simulink library "Adaptive_FaultTolerantControl"  (R2015a)
settings: Solver=ode45  StartTime=0.0  StopTime=10.0  RelTol=1e-3
libraries: qcatlib x1
settings Model: Creator=David  LastModifiedBy=David
settings OptimizationCC: ExpressionDepthLimit=2147483647
settings DebuggingCC: UnderspecifiedInitializationDetection=Classic  MergeDetectMultiDrivingBlocksExec=none  SolverPrmCheckMsg=warning  StateNameClashWarn=warning

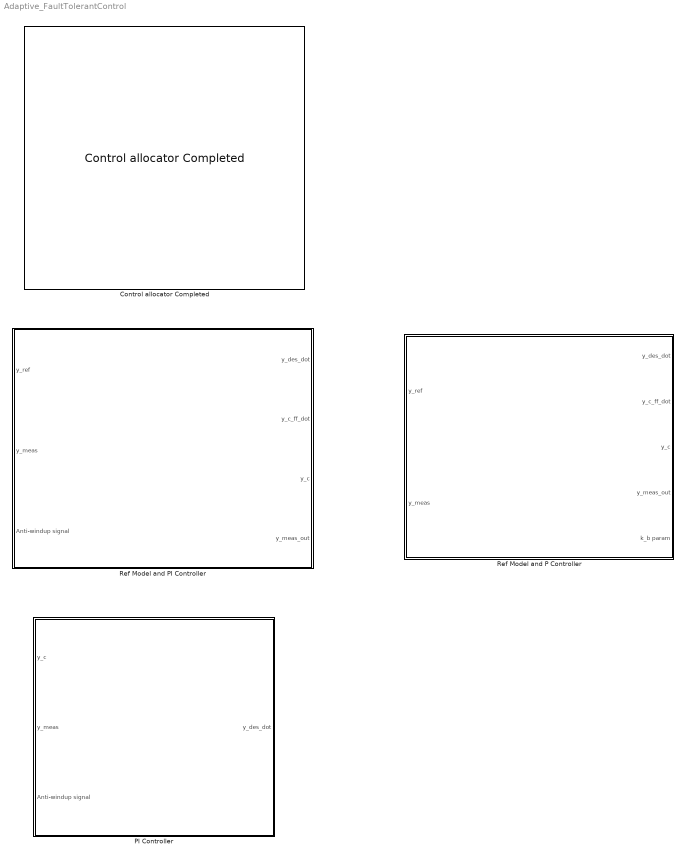
== system Adaptive_FaultTolerantControl ==
  "Control allocator Completed " : qcatlib/Control allocator Completed   alg=WLS  CA_type=DYN  iter_max=100  gamma=1e6  k_B=3  m_B=7  T=0.01  tol=0
  PI Controller : Subsystem  mask(PI Controller){delta=0, K_a=0, y_i=0, Des_way=auto, omega_n=10, xi=0.9, Z1=0, K_b=12, f_i=0.25, f_c=1}
      mask prompts: delta "Integrator delay"; K_a "Anti-windup gain"; y_i "Initial state"; Des_way "Expected response: Controller Design process"; omega_n "Desired 2nd order response omega_n"; xi "Desired 2nd order response  xi"; Z1 "Zero of controller"; K_b "K_b proportional term"; f_i "f_i integral term"; f_c "f_c fedfordward term (1 recomended)"
      mask help:
      | Author David Torres
      | This bock generates a desired rate for an error inputa y_c-y_meas
      |
      | I also include antiwind up and feedforward signal
      mask init:
      | val = get_param(gcb,'MaskValues');
      | % Controller design
      | switch lower(val{4})
      |     case 'auto'
      |         K_b=2*xi*omega_n;
      |         f_i=1/(4*xi^2);
      |         if f_i<0.25
      |             f_c = 0.5*(1+sqrt(1-4*f_i));
      |         else
      |             f_c = sqrt(f_i);
      |         end
      |     case 'advanced'
      |         K_b=2*xi*omega_n;
      |         f_i=1/(4*xi^2);
      |         f_c =  -omega_n/(2*xi*Z1);  
      |     case 'pro'
      | end
      mask TypeOptions Des_way: auto | advanced | pro
      mask Callback Des_way:
      | val = get_param(gcb,'MaskValues');
      | switch lower(val{4})
      |     case 'auto'
      |         set_param(gcb,'MaskVisibilities',{'on','on','on','on','on','on','off','off','off','off'});
      |     case 'advanced'
      |         set_param(gcb,'MaskVisibilities',{'on','on','on','on','on','on','on','off','off','off'});
      |     case 'pro'
      |         set_param(gcb,'MaskVisibilities',{'on','on','on','on','off','off','off','on','on','on'});
      |  end
      mask Display:
      | if delta==0
      |     TF = tf(K_b*[f_c f_i*K_b],[1 K_b f_i*K_b^2]);
      | else
      |     s=tf('s');
      |     TF = 1/(s+delta)*K_b*(f_c*s+f_i*K_b)/(s*( 1+1/(s+delta)*K_b ) + 1/(s+delta)*f_i*K_b^2 );
      | end
      | 
      | [y,t]=step(TF);
      | S = stepinfo(y,t);
      | 
      | pos = get_param(gcb, 'Position');
      | width = pos(3) - pos(1);
      | height = pos(4) - pos(2);
      | t = t.*width/max(t);
      | y=y.*height/max(y);
      | plot(t,y);
      | 
      | S2 = stepinfo(y,t);
      | if S2.PeakTime<0.5*width
      |     Peaktime = S2.PeakTime;
      | else
      |     Peaktime = 0.25*width;
      | end
      | text(Peaktime ,S2.Peak*0.85,['Peak time = ',num2str(S.PeakTime),'s' ]);
      | text(Peaktime ,S2.Peak*0.75,['Os = ',num2str(S.Peak)]);
      | text(Peaktime ,S2.Peak*0.75,['Os = ',num2str(S.Peak)]);
      | text(Peaktime ,S2.Peak*0.65,['SettlingTime = ',num2str(S.SettlingTime)]);
      | 
      | text(0.05*width,0.1*height,['EXPECTED CLOSED-LOOP RESPONSE: INTEGRATION DELAY ',num2str(delta),'s ']);
      | 
      | [num,den] = tfdata(TF);
      | dpoly(num{:},den{:}, 's');
  Ref Model and P Controller : Subsystem  mask(Reference Model and Controller){tau=0.2, y_i=0, K_f=1, K_b=1}
      mask prompts: tau "Desired time constant tau"; y_i "Initial state"; K_f "Rate Feedfordward Gain K_f"; K_b "Proportional Gain K_b"
      mask help:
      | Author: David Torres
      |
      | This block allows a design of the desired dynamics as a 1st order system and the controller of it with P and I actions, with feedforward in rate and anti-windup action.
      |
      |     Inputs: Signal reference, Signal measurement and anti-windup dignal.
      |     Outputs: Desired Signal rate
      |
      | The block shows the expected dynamics assuming the output is integrated with a PERFECT INTEGRATOR or an INTEGRATOR WITH DELAY(delta):
      |      NDI, CA and plant act as a perfect integrator or integrator with a delay delta.
      mask TypeOptions tau: Reference Model/tau
      mask TypeOptions y_i: Reference Model/y_i
      mask TypeOptions K_f: K_f/Gain
      mask TypeOptions K_b: K_b params/Value
      mask Display:
      | K_ref=1/tau;
      | TF = tf([K_ref],[1 K_ref]);
      | 
      | [y,t]=step(TF);
      | S = stepinfo(y,t);
      | 
      | pos = get_param(gcb, 'Position');
      | width = pos(3) - pos(1);
      | height = pos(4) - pos(2);
      | t = t.*width/max(t);
      | y=y.*height/max(y);
      | plot(t,y);
      | S2 = stepinfo(y,t);
      | 
      | if S.Overshoot==0 % 1st order response
      |     text(S2.RiseTime ,height*0.85,['Rise time = ',num2str(S.RiseTime),'s' ]);
      |     text(S2.RiseTime ,height*0.75,['Settling Time = ',num2str(S.SettlingTime)]);
      | 
      | elseif S.Overshoot<0.05 % 2nd order response
      |     text(width*0.5 ,height*0.9,['Rise time = ',num2str(S.RiseTime),'s' ]);
      |     text(width*0.5 ,height*0.8,['Pike time = ',num2str(S.PeakTime),'s' ]);
      |     text(width*0.5 ,height*0.7,['Os = ',num2str(S.Peak)]);
      |     text(width*0.5 ,height*0.6,['SettlingTime = ',num2str(S.SettlingTime)]);
      | else % 2nd order response
      |     text(S2.PeakTime ,S2.Peak*0.85,['Peak time = ',num2str(S.PeakTime),'s' ]);
      |     text(S2.PeakTime ,S2.Peak*0.75,['Os = ',num2str(S.Peak)]);
      |     text(S2.PeakTime ,S2.Peak*0.65,['SettlingTime = ',num2str(S.SettlingTime)]);
      | end
      | 
      | 
      | [num,den] = tfdata(TF);
      | dpoly(num{:},den{:}, 's');
  Ref Model and PI Controller : Subsystem  mask(Reference Model and Controller){delta=0, tau=0.5, y_i=0, K_f=1, K_a=1, Con_way=auto, omega_n=4, xi=0.5, Z1=-30, K_b=2*0.8*3, f_i=0.25*1/0.8^2, f_c=1}
      mask prompts: delta "Delay on assumed integration: delta (0 for ideal integration)"; tau "Desired time constant tau"; y_i "Initial state"; K_f "Rate Feedfordward Gain"; K_a "Anti-windup gain K_a"; Con_way "Expected response: Controller Design process"; omega_n "Desired 2nd order response omega_n"; xi "Desired 2nd order response  xi"; Z1 "Zero of controller"
      mask help:
      | Author: David Torres
      |
      | This block allows a design of the desired dynamics as a 1st order system and the controller of it with P and I actions, with feedforward in rate and anti-windup action.
      |
      |     Inputs: Signal reference, Signal measurement and anti-windup dignal.
      |     Outputs: Desired Signal rate
      |
      | The block shows the expected dynamics assuming the output is integrated with a PERFECT INTEGRATOR or an INTEGRATOR WITH DELAY(delta):
      |      NDI, CA and plant act as a perfect integrator or integrator with a delay delta.
      mask init:
      | val = get_param(gcb,'MaskValues');
      | K_ref=1/tau;	
      | % Controller design
      | switch lower(val{6})
      |     case 'auto'
      |         K_b=2*xi*omega_n;
      |         f_i=1/(4*xi^2);
      |         if f_i<0.25
      |             f_c = 0.5*(1+sqrt(1-4*f_i));
      |         else
      |             f_c = sqrt(f_i);
      |         end
      |     case 'advanced'
      |         K_b=2*xi*omega_n;
      |         f_i=1/(4*xi^2);
      |         f_c =  -omega_n/(2*xi*Z1);  
      |     case 'pro'
      | end
      mask TypeOptions delta: PI Controller/delta
      mask TypeOptions tau: Reference Model/tau
      mask TypeOptions y_i: Reference Model/y_i
      mask TypeOptions K_f: K_f/Gain
      mask TypeOptions K_a: PI Controller/K_a
      mask TypeOptions Con_way: auto | advanced | pro
      mask Callback Con_way:
      | val = get_param(gcb,'MaskValues');
      | switch lower(val{6})
      |  case 'auto'
      |      set_param(gcb,'MaskVisibilities',{'on','on','on','on','on','on','on','on','off','off','off','off'});
      |  case 'advanced'
      |      set_param(gcb,'MaskVisibilities',{'on','on','on','on','on','on','on','on','on','off','off','off'});
      |  case 'pro'
      |      set_param(gcb,'MaskVisibilities',{'on','on','on','on','on','on','off','off','off','on','on','on'});
      |  end
      mask TypeOptions K_b: PI Controller/K_b
      mask TypeOptions f_i: PI Controller/f_i
      mask TypeOptions f_c: PI Controller/f_c
      mask Display:
      | RM = tf([K_ref],[1 K_ref]);
      | 
      | if delta==0
      |     TF_FF = tf([K_f K_b*f_c K_b*f_i*K_b],[1 K_b f_i*K_b^2]);
      | else
      |     s=tf('s');
      |     TF_FF = 1/(s+delta)*(K_f*s^2+K_b*(f_c*s+f_i*K_b))/(s + 1/(s+delta)*(K_b*s+f_i*K_b^2) );
      | end
      | TF = RM*TF_FF;
      | 
      | [y,t]=step(TF);
      | S = stepinfo(y,t);
      | 
      | pos = get_param(gcb, 'Position');
      | width = pos(3) - pos(1);
      | height = pos(4) - pos(2);
      | t = t.*width/max(t);
      | y=y.*height/max(y);
      | plot(t,y);
      | S2 = stepinfo(y,t);
      | 
      | if S.Overshoot==0 % 1st order response
      |     text(S2.RiseTime ,height*0.85,['Rise time = ',num2str(S.RiseTime),'s' ]);
      |     text(S2.RiseTime ,height*0.75,['Settling Time = ',num2str(S.SettlingTime)]);
      | 
      | elseif S.Overshoot<0.05 % 2nd order response
      |     text(width*0.5 ,height*0.9,['Rise time = ',num2str(S.RiseTime),'s' ]);
      |     text(width*0.5 ,height*0.8,['Pike time = ',num2str(S.PeakTime),'s' ]);
      |     text(width*0.5 ,height*0.7,['Os = ',num2str(S.Peak)]);
      |     text(width*0.5 ,height*0.6,['SettlingTime = ',num2str(S.SettlingTime)]);
      | else % 2nd order response
      |     text(S2.PeakTime ,S2.Peak*0.85,['Peak time = ',num2str(S.PeakTime),'s' ]);
      |     text(S2.PeakTime ,S2.Peak*0.75,['Os = ',num2str(S.Peak)]);
      |     text(S2.PeakTime ,S2.Peak*0.65,['SettlingTime = ',num2str(S.SettlingTime)]);
      | end
      | 
      | text(0.1*width,0.1*height,['EXPECTED CLOSED-LOOP RESPONSE: INTEGRATION DELAY OF ',num2str(delta),'s ']);
      | 
      | [num,den] = tfdata(TF);
      | dpoly(num{:},den{:}, 's');

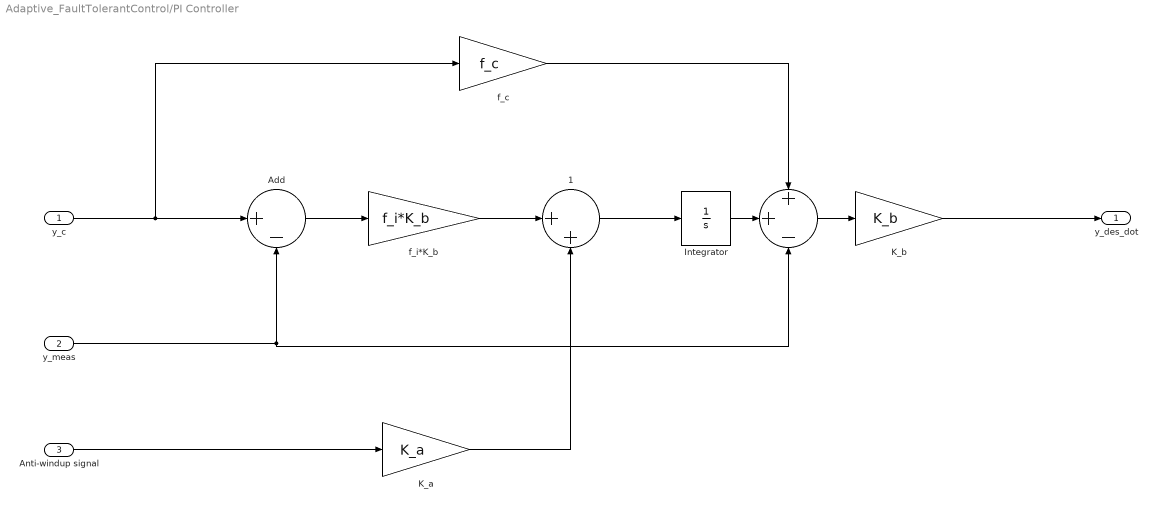
== system Adaptive_FaultTolerantControl/PI Controller ==
  y_c : Inport
  y_meas : Inport  Port=2
  Anti-windup signal : Inport  Port=3
  " " : Sum  Inputs=++-
  " 1" : Sum  Inputs=|++
  Add : Sum  Inputs=|+-
  Integrator : Integrator  InitialCondition=y_i*(1-f_c)
  K_a : Gain  Gain=K_a
  K_b : Gain  Gain=K_b
  f_c : Gain  Gain=f_c
  f_i*K_b : Gain  Gain=f_i*K_b
  y_des_dot : Outport
  wires:
  f_i*K_b/1 -> " 1"/1
  Add/1 -> f_i*K_b/1
  K_b/1 -> y_des_dot/1
  y_meas/1 -> Add/2, " "/3
  y_c/1 -> f_c/1, Add/1
  Integrator/1 -> " "/2
  f_c/1 -> " "/1
  " "/1 -> K_b/1
  Anti-windup signal/1 -> K_a/1
  " 1"/1 -> Integrator/1
  K_a/1 -> " 1"/2

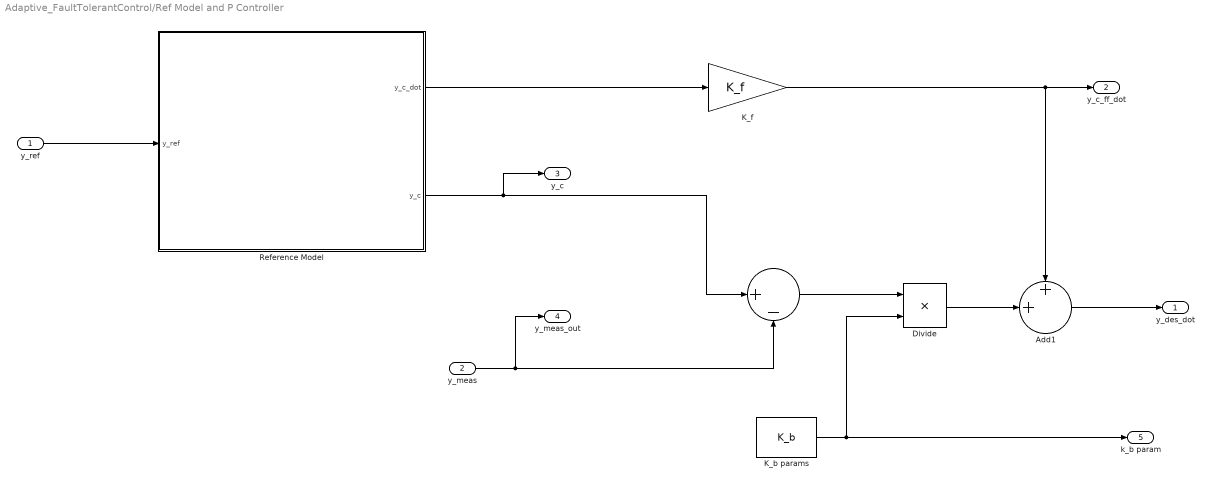
== system Adaptive_FaultTolerantControl/Ref Model and P Controller ==
  y_ref : Inport
  y_meas : Inport  Port=2
  " " : Sum  Inputs=|+-
  Add1 : Sum  Inputs=++|
  Divide : Product  Inputs=**
  K_b params : Constant  Value=K_b
  K_f : Gain  Gain=K_f
  Reference Model : Subsystem  mask{tau=tau, y_i=y_i}
      mask prompts: tau "1st order time constant (tau)"; y_i "Initial state"
      mask init:
      | K_ref=1/tau;
      mask Display:
      | [y,t]=step(tf([K_ref],[1 K_ref]));
      | pos = get_param(gcb, 'Position');
      | width = pos(3) - pos(1);
      | height = pos(4) - pos(2);
      | t = t.*width/max(t);
      | y=y.*height/max(y);
      | plot(t,y);
      | 
      | 
      | text(0.5*width,0.92*height,['tau=',num2str(tau)]);
      | 
      | dpoly([K_ref],[1 K_ref], 's')
  y_des_dot : Outport
  y_c_ff_dot : Outport  Port=2
  y_c : Outport  Port=3
  y_meas_out : Outport  Port=4
  k_b param : Outport  Port=5
  wires:
  Divide/1 -> Add1/2
  K_f/1 -> Add1/1, y_c_ff_dot/1
  Reference Model/1(y_c_dot) -> K_f/1
  Add1/1 -> y_des_dot/1
  y_ref/1 -> Reference Model/1(y_ref)
  " "/1 -> Divide/1
  Reference Model/2(y_c) -> " "/1, y_c/1
  y_meas/1 -> " "/2, y_meas_out/1
  K_b params/1 -> Divide/2, k_b param/1

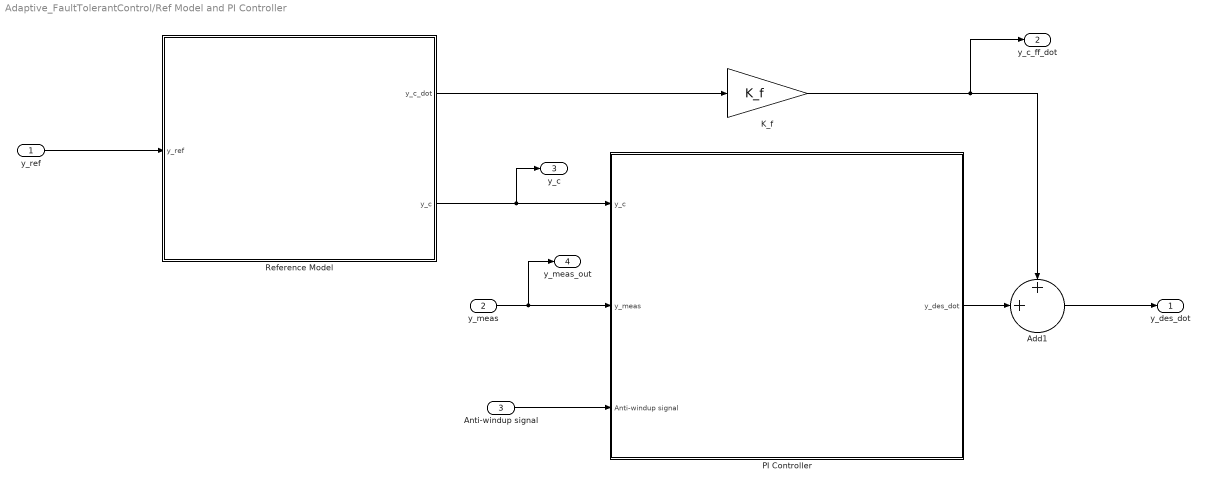
== system Adaptive_FaultTolerantControl/Ref Model and PI Controller ==
  y_ref : Inport
  y_meas : Inport  Port=2
  Anti-windup signal : Inport  Port=3
  Add1 : Sum  Inputs=++|
  K_f : Gain  Gain=K_f
  PI Controller : Subsystem  mask{K_b=K_b, f_i=f_i, f_c=f_c, K_a=K_a, delta=delta}
      mask prompts: K_b "K_b proportional term"; f_i "f_i integral term"; f_c "f_c fedfordward term"; K_a "Anti-windup gain"; delta "Integrator delay"
      mask Display:
      | if delta==0
      |     TF = tf(K_b*[f_c f_i*K_b],[1 K_b f_i*K_b^2]);
      | else
      |     s=tf('s');
      |     TF = 1/(s+delta)*K_b*(f_c*s+f_i*K_b)/(s*( 1+1/(s+delta)*K_b ) + 1/(s+delta)*f_i*K_b^2 );
      | end
      | 
      | [y,t]=step(TF);
      | S = stepinfo(y,t);
      | 
      | pos = get_param(gcb, 'Position');
      | width = pos(3) - pos(1);
      | height = pos(4) - pos(2);
      | t = t.*width/max(t);
      | y=y.*height/max(y);
      | plot(t,y);
      | 
      | S2 = stepinfo(y,t);
      | text(S2.PeakTime ,S2.Peak*0.85,['Peak time = ',num2str(S.PeakTime),'s' ]);
      | text(S2.PeakTime ,S2.Peak*0.75,['Os = ',num2str(S.Peak)]);
      | text(S2.PeakTime ,S2.Peak*0.75,['Os = ',num2str(S.Peak)]);
      | text(S2.PeakTime ,S2.Peak*0.65,['SettlingTime = ',num2str(S.SettlingTime)]);
      | 
      | text(0.1*width,0.1*height,['EXPECTED CLOSED-LOOP RESPONSE: INTEGRATION DELAY OF ',num2str(delta),'s ']);
      | 
      | [num,den] = tfdata(TF);
      | dpoly(num{:},den{:}, 's');
  Reference Model : Subsystem  mask{tau=tau, y_i=y_i}
      mask prompts: tau "1st order time constant (tau)"; y_i "Initial state"
      mask init:
      | K_ref=1/tau;
      mask Display:
      | [y,t]=step(tf([K_ref],[1 K_ref]));
      | pos = get_param(gcb, 'Position');
      | width = pos(3) - pos(1);
      | height = pos(4) - pos(2);
      | t = t.*width/max(t);
      | y=y.*height/max(y);
      | plot(t,y);
      | 
      | 
      | text(0.5*width,0.92*height,['tau=',num2str(tau)]);
      | 
      | dpoly([K_ref],[1 K_ref], 's')
  y_des_dot : Outport
  y_c_ff_dot : Outport  Port=2
  y_c : Outport  Port=3
  y_meas_out : Outport  Port=4
  wires:
  y_ref/1 -> Reference Model/1(y_ref)
  Reference Model/2(y_c) -> y_c/1, PI Controller/1(y_c)
  Add1/1 -> y_des_dot/1
  Reference Model/1(y_c_dot) -> K_f/1
  K_f/1 -> y_c_ff_dot/1, Add1/1
  PI Controller/1(y_des_dot) -> Add1/2
  Anti-windup signal/1 -> PI Controller/3(Anti-windup signal)
  y_meas/1 -> y_meas_out/1, PI Controller/2(y_meas)

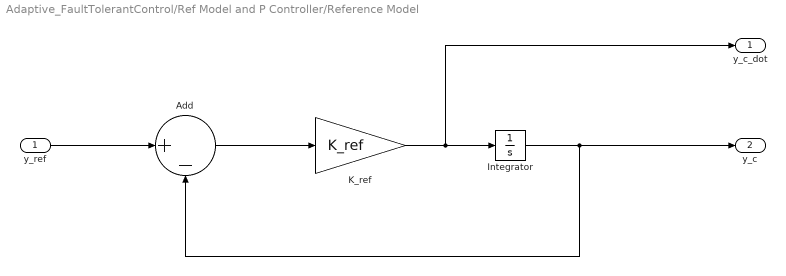
== system Adaptive_FaultTolerantControl/Ref Model and P Controller/Reference Model ==
  y_ref : Inport
  Add : Sum  Inputs=|+-
  Integrator : Integrator  InitialCondition=y_i
  K_ref : Gain  Gain=K_ref
  y_c_dot : Outport
  y_c : Outport  Port=2
  wires:
  Integrator/1 -> Add/2, y_c/1
  K_ref/1 -> y_c_dot/1, Integrator/1
  Add/1 -> K_ref/1
  y_ref/1 -> Add/1

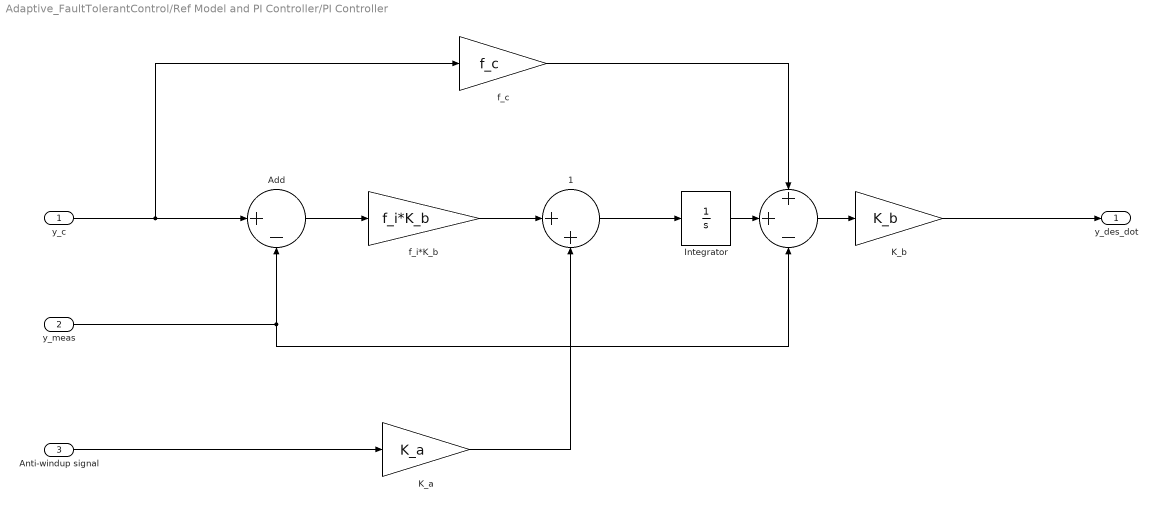
== system Adaptive_FaultTolerantControl/Ref Model and PI Controller/PI Controller ==
  y_c : Inport
  y_meas : Inport  Port=2
  Anti-windup signal : Inport  Port=3
  " " : Sum  Inputs=++-
  " 1" : Sum  Inputs=|++
  Add : Sum  Inputs=|+-
  Integrator : Integrator
  K_a : Gain  Gain=K_a
  K_b : Gain  Gain=K_b
  f_c : Gain  Gain=f_c
  f_i*K_b : Gain  Gain=f_i*K_b
  y_des_dot : Outport
  wires:
  f_i*K_b/1 -> " 1"/1
  Add/1 -> f_i*K_b/1
  K_b/1 -> y_des_dot/1
  y_meas/1 -> " "/3, Add/2
  y_c/1 -> f_c/1, Add/1
  Integrator/1 -> " "/2
  f_c/1 -> " "/1
  " "/1 -> K_b/1
  Anti-windup signal/1 -> K_a/1
  " 1"/1 -> Integrator/1
  K_a/1 -> " 1"/2

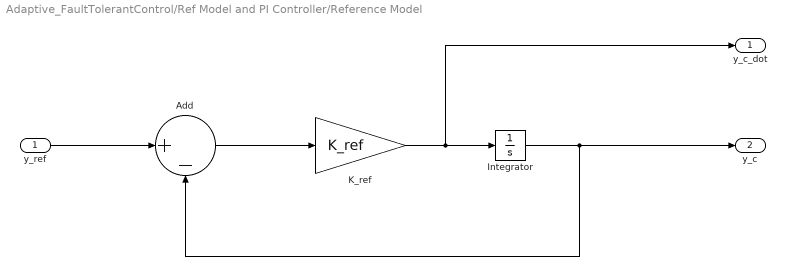
== system Adaptive_FaultTolerantControl/Ref Model and PI Controller/Reference Model ==
  y_ref : Inport
  Add : Sum  Inputs=|+-
  Integrator : Integrator  InitialCondition=y_i
  K_ref : Gain  Gain=K_ref
  y_c_dot : Outport
  y_c : Outport  Port=2
  wires:
  y_ref/1 -> Add/1
  Add/1 -> K_ref/1
  K_ref/1 -> Integrator/1, y_c_dot/1
  Integrator/1 -> y_c/1, Add/2
